simulink model "sim_lowpass"  (Simulink 8.5)
settings: Solver=ode3  StartTime=0.0  StopTime=5  FixedStep=0.01  RelTol=1e-3
settings Model: Creator=sifi  LastModifiedBy=sifi
settings DataIOCC: SignalLoggingSaveFormat=Dataset
settings OptimizationCC: ExpressionDepthLimit=128
settings DebuggingCC: UnderspecifiedInitializationDetection=Simplified  MergeDetectMultiDrivingBlocksExec=error  FcnCallInpInsideContextMsg=EnableAllAsError  StateNameClashWarn=none
settings GRTTargetCC: CombineOutputUpdateFcns=on  GRTInterface=off

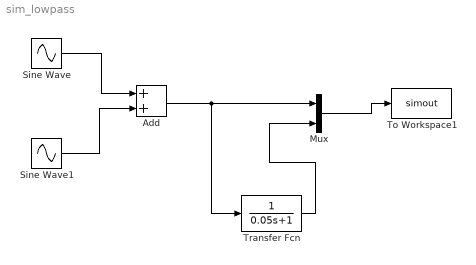
== system sim_lowpass ==
  Add : Sum
  Mux : Mux  Inputs=2
  Sine Wave : Sin  Amplitude=1.5  Frequency=2*pi/3  SampleTime=0
  Sine Wave1 : Sin  Frequency=40*pi  SampleTime=0
  To Workspace1 : ToWorkspace  VariableName=simout  SampleTime=-1
  Transfer Fcn : TransferFcn  Denominator=[0.05 1]
  wires:
  Sine Wave/1 -> Add/1
  Sine Wave1/1 -> Add/2
  Transfer Fcn/1 -> Mux/2
  Add/1 -> Mux/1, Transfer Fcn/1
  Mux/1 -> To Workspace1/1
